simulink model "actividad1"  (R2020a)
settings: Solver=VariableStepAuto  StartTime=0.0  StopTime=10.0  RelTol=1e-3
settings Model: Creator=xsraj  LastModifiedBy=xsraj

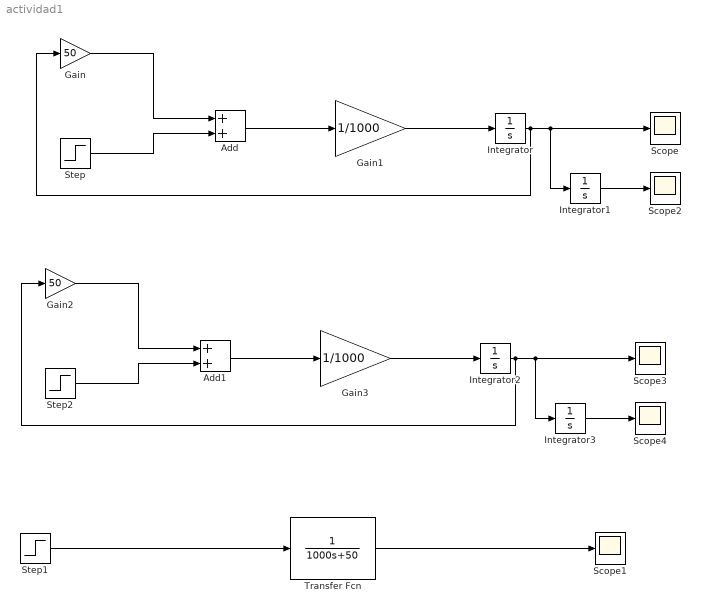
== system actividad1 ==
  Add : Sum
  Add1 : Sum
  Gain : Gain  Gain=50
  Gain1 : Gain  Gain=1/1000
  Gain2 : Gain  Gain=50
  Gain3 : Gain  Gain=1/1000
  Integrator{,1..3} (4 alike) : Integrator
  Scope{,1..4} (5 alike) : Scope
  Step : Step  SampleTime=0
  Step1 : Step  SampleTime=0
  Step2 : Step  SampleTime=0
  Transfer Fcn : TransferFcn  Denominator=[1000 50]
  wires:
  Step/1 -> Add/2
  Gain/1 -> Add/1
  Integrator/1 -> Integrator1/1, Scope/1, Gain/1
  Add/1 -> Gain1/1
  Gain1/1 -> Integrator/1
  Step1/1 -> Transfer Fcn/1
  Transfer Fcn/1 -> Scope1/1
  Integrator1/1 -> Scope2/1
  Gain3/1 -> Integrator2/1
  Add1/1 -> Gain3/1
  Integrator2/1 -> Integrator3/1, Scope3/1, Gain2/1
  Gain2/1 -> Add1/1
  Step2/1 -> Add1/2
  Integrator3/1 -> Scope4/1
